simulink model "Compensador_RLC"  (R2015a)
settings: Solver=ode45  StartTime=0.0  StopTime=10.0  RelTol=1e-3
values from neighbouring files (symbols this model uses):
  C1 = 0.22    [Compensador_Adelanto.m]    (also in Compensador_Atraso.m = 0.0001)
  C2 = 0.010    (= 0.01)    [Compensador_Adelanto.m]    (also in Compensador_Atraso.m = 0.002)
  R1 = 3900    [Compensador_Adelanto.m]    (also in Compensador_Atraso.m = 2200)
  R2 = 1800    [Compensador_Adelanto.m]    (also in Compensador_Atraso.m = 3300)
  R3 = 2700    [Compensador_Adelanto.m]    (also in Compensador_Atraso.m = 1500)
  R4 = 4700    [Compensador_Adelanto.m]    (also in Compensador_Atraso.m)
libraries: slctrlblks x1
settings Model: Creator=Henry Alberto  LastModifiedBy=Henry Alberto

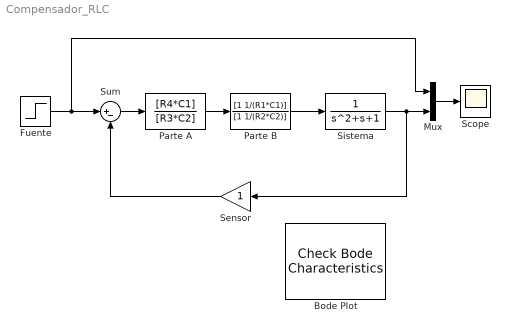
== system Compensador_RLC ==
  Bode Plot : slctrlblks/Model Verification/Check Bode  Characteristics  InstantiateOnLoad=on  SaveOperatingPoints=off  LinearizationIOs={}  LinearizeAt=SnapshotTimes  SnapshotTimes=[0]  TriggerType=rising  SampleTime=auto  RateConversionMethod=zoh  PreWarpFreq=10  UseExactDelayModel=off  UseFullBlockNameLabels=off  UseBusSignalLabels=off  enabled=on  stopWhenAssertionFail=off  export=off  ViewDlgPos=[]  OpenViewOnLoad=off  LaunchViewOnOpen=off  FrequencyUnits=rad/s  MagnitudeUnits=dB  PhaseUnits=deg  TimeUnits=seconds  EnableUpperBound=off  UpperBoundFrequencies=[]  UpperBoundMagnitudes=[]  EnableLowerBound=off  LowerBoundFrequencies=[]  LowerBoundMagnitudes=[]
  Fuente : Step  SampleTime=0
  Mux : Mux  Inputs=2
  Parte A : TransferFcn  Numerator=[R4*C1]  Denominator=[R3*C2]
  Parte B : TransferFcn  Numerator=[1 1/(R1*C1)]  Denominator=[1 1/(R2*C2)]
  Scope : Scope
  Sensor : Gain
  Sistema : TransferFcn  Denominator=[1 1 1]
  Sum : Sum  Inputs=|+-
  wires:
  Sistema/1 -> Mux/2, Sensor/1
  Fuente/1 -> Sum/1, Mux/1
  Sensor/1 -> Sum/2
  Mux/1 -> Scope/1
  Sum/1 -> Parte A/1
  Parte A/1 -> Parte B/1
  Parte B/1 -> Sistema/1
